simulink model "simulation_eolienne"  (R2021b)
settings: Solver=VariableStepAuto  StartTime=0.0  StopTime=120  RelTol=1e-3
values from neighbouring files (symbols this model uses):
  sys = ss(A,[B Bd],C,zeros(1,3))    [Init_Parametres_Eolienne.m]
settings Model: Creator=Rodriguez  LastModifiedBy=Rodriguez

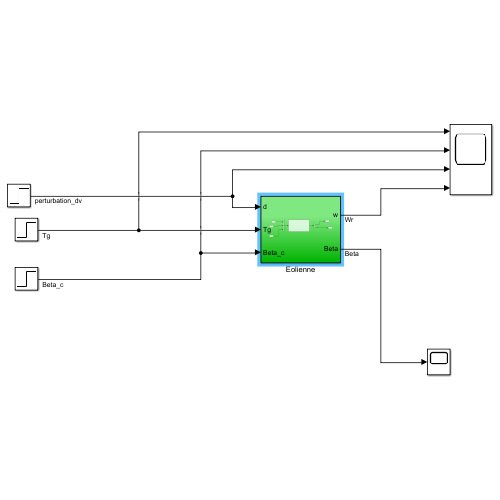
[thumbnail: Simulink's stored preview of the top-level diagram]
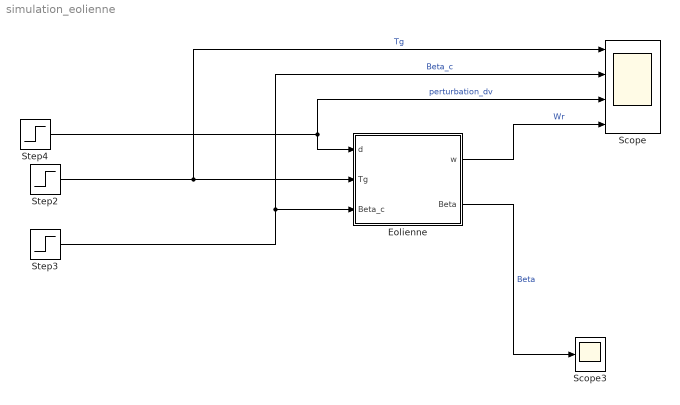
== system simulation_eolienne ==
  Eolienne : Subsystem
  Scope : Scope  NumInputPorts=4
  Scope3 : Scope
  Step2 : Step  Time=10  After=10000  SampleTime=0
  Step3 : Step  Time=50  SampleTime=0
  Step4 : Step  Time=80  SampleTime=0
  wires:
  Eolienne/1(w) -> Scope/4  "Wr"
  Step2/1 -> Eolienne/2(Tg), Scope/1  "Tg"
  Step3/1 -> Eolienne/3(Beta_c), Scope/2  "Beta_c"
  Step4/1 -> Eolienne/1(d), Scope/3  "perturbation_dv"
  Eolienne/2(Beta) -> Scope3/1  "Beta"

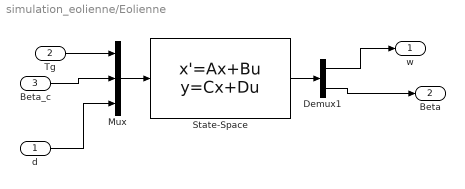
== system simulation_eolienne/Eolienne ==
  d : Inport
  Tg : Inport  Port=2
  Beta_c : Inport  Port=3
  Demux1 : Demux  Outputs=2
  Mux : Mux  Inputs=3
  State-Space : StateSpace  A=sys.a  B=sys.b  C=eye(2)  D=zeros(2,3)  InitialCondition=0
  w : Outport
  Beta : Outport  Port=2
  wires:
  State-Space/1 -> Demux1/1
  Mux/1 -> State-Space/1
  Tg/1 -> Mux/1
  d/1 -> Mux/3
  Demux1/1 -> w/1
  Demux1/2 -> Beta/1
  Beta_c/1 -> Mux/2
